simulink model "RADTRANS001"  (R2020b)
settings: Solver=VariableStepAuto  StartTime=0.0  StopTime=10.0  RelTol=1e-3
undefined symbols (not defined in the file): Line_110_C, Line_110_L, Line_110_R, Line_220_C, Line_220_L, Line_220_R, Line_35_C, Line_35_L, Line_35_R, Line_6_L, Line_6_R, Sys_f_Hz, Sys_V_net_kV, Tr_110_35_L_pu, Tr_110_35_R_pu, Tr_110_35_Sn_VA, Tr_110_35_V_HV_kV, Tr_110_35_V_LV_kV, Tr_110_6_L_pu, Tr_110_6_R_pu, Tr_110_6_Sn_VA, Tr_110_6_V_HV_kV, Tr_110_6_V_LV_kV, Tr_220_110_L_pu, Tr_220_110_R_pu, Tr_220_110_Sn_VA, Tr_220_110_V_HV_kV, Tr_220_110_V_LV_kV, Tr_35_04_L_pu, Tr_35_04_R_pu, Tr_35_04_Sn_VA, Tr_35_04_V_HV_kV, Tr_35_04_V_LV_kV, Tr_6_04_L_pu, Tr_6_04_R_pu, Tr_6_04_Sn_VA, Tr_6_04_V_HV_kV, Tr_6_04_V_LV_kV, Ts_powergui
libraries: dspstat3 x240, powerlib x169, powerlib_meascontrol x60
(part 6 of 6)

== system RADTRANS001/M_OUT_Завод_1_2 ==
  Iptg_4 : Display
      settings: Format=bank
  PQptg_4 : Scope  NumInputPorts=2
  "Power0 (3ph, Instantaneous)" : powerlib_meascontrol/Measurements/Power (3ph, Instantaneous)
  Pptg_4 : Display
      settings: Format=bank
  Qptg_4 : Display
      settings: Format=bank
  RMS0 : dspstat3/RMS  run=off  directionMode=Each column  dimension=1  InputProcessing=Columns as channels (frame based)  reset_popup=None
  RMS3 : dspstat3/RMS  run=off  directionMode=Each column  dimension=1  InputProcessing=Columns as channels (frame based)  reset_popup=None
  RMS4 : dspstat3/RMS  run=off  directionMode=Each column  dimension=1  InputProcessing=Columns as channels (frame based)  reset_popup=None
  RMSpt_4 : dspstat3/RMS  run=off  directionMode=Each column  dimension=1  InputProcessing=Columns as channels (frame based)  reset_popup=None
  Real-Ima to Complex : RealImagToComplex
  S : Abs
  SSptg_4 : Scope
  Sptg_4 : Display
      settings: Format=bank
  Three-Phase V-I Measurementpt_4 : powerlib/Measurements/Three-Phase V-I Measurement  VoltageMeasurement=phase-to-ground  SetLabelV=off  LabelV=Vabc  Vpu=off  VpuLL=off  CurrentMeasurement=yes  SetLabelI=off  LabelI=Iabc  Ipu=off  Pbase=100e6  Vbase=500e3  OutputType=Complex  PhasorSimulation=off  PSBequivalent=0
  UIptg_4 : Scope  NumInputPorts=2
  Uptg_4 : Display
      settings: Format=bank
  a : PMIOPort  Side=Right
  b : PMIOPort  Port=2  Side=Right
  c : PMIOPort  Port=3  Side=Right
  A : PMIOPort  Port=4  Side=Left
  B : PMIOPort  Port=5  Side=Left
  C : PMIOPort  Port=6  Side=Left
  tag scope: I_ptg_4=global, P_ptg_4=global, Q_ptg_4=global, S_ptg_4=global, U_ptg_4=global
  wires:
  S/1 -> [S_ptg_4]
  Real-Ima to Complex/1 -> S/1
  [S_ptg_4] -> Sptg_4/1
  [S_ptg_4] -> SSptg_4/1
  [P_ptg_4] -> RMSpt_4/1
  RMSpt_4/1 -> Pptg_4/1
  RMS0/1 -> Qptg_4/1
  [U_ptg_4] -> RMS3/1
  RMS3/1 -> Uptg_4/1
  [P_ptg_4] -> Real-Ima to Complex/1
  [Q_ptg_4] -> RMS0/1
  [I_ptg_4] -> RMS4/1
  RMS4/1 -> Iptg_4/1
  [U_ptg_4] -> UIptg_4/1  "U"
  [P_ptg_4] -> PQptg_4/1  "P"
  [I_ptg_4] -> UIptg_4/2  "I"
  Three-Phase V-I Measurementpt_4/1 -> [U_ptg_4]
  [Q_ptg_4] -> Real-Ima to Complex/2
  Three-Phase V-I Measurementpt_4/2 -> [I_ptg_4]
  [U_ptg_4] -> "Power0 (3ph, Instantaneous)"/1
  [I_ptg_4] -> "Power0 (3ph, Instantaneous)"/2
  "Power0 (3ph, Instantaneous)"/2 -> [Q_ptg_4]
  "Power0 (3ph, Instantaneous)"/1 -> [P_ptg_4]
  [Q_ptg_4] -> PQptg_4/2  "Q"
  connections:
  Three-Phase V-I Measurementpt_4/LConn1 -- A/RConn1
  Three-Phase V-I Measurementpt_4/RConn1 -- a/RConn1
  Three-Phase V-I Measurementpt_4/LConn2 -- B/RConn1
  Three-Phase V-I Measurementpt_4/LConn3 -- C/RConn1
  Three-Phase V-I Measurementpt_4/RConn3 -- c/RConn1
  Three-Phase V-I Measurementpt_4/RConn2 -- b/RConn1

== system RADTRANS001/M_OUT_Завод_2_1 ==
  Iptg_14 : Display
      settings: Format=bank
  PQptg_14 : Scope  NumInputPorts=2
  "Power0 (3ph, Instantaneous)" : powerlib_meascontrol/Measurements/Power (3ph, Instantaneous)
  Pptg_14 : Display
      settings: Format=bank
  Qptg_14 : Display
      settings: Format=bank
  RMS14 : dspstat3/RMS  run=off  directionMode=Each column  dimension=1  InputProcessing=Columns as channels (frame based)  reset_popup=None
  RMS3 : dspstat3/RMS  run=off  directionMode=Each column  dimension=1  InputProcessing=Columns as channels (frame based)  reset_popup=None
  RMS4 : dspstat3/RMS  run=off  directionMode=Each column  dimension=1  InputProcessing=Columns as channels (frame based)  reset_popup=None
  RMSpt_14 : dspstat3/RMS  run=off  directionMode=Each column  dimension=1  InputProcessing=Columns as channels (frame based)  reset_popup=None
  Real-Ima to Complex : RealImagToComplex
  S : Abs
  SSptg_14 : Scope
  Sptg_14 : Display
      settings: Format=bank
  Three-Phase V-I Measurementpt_14 : powerlib/Measurements/Three-Phase V-I Measurement  VoltageMeasurement=phase-to-ground  SetLabelV=off  LabelV=Vabc  Vpu=off  VpuLL=off  CurrentMeasurement=yes  SetLabelI=off  LabelI=Iabc  Ipu=off  Pbase=100e6  Vbase=500e3  OutputType=Complex  PhasorSimulation=off  PSBequivalent=0
  UIptg_14 : Scope  NumInputPorts=2
  Uptg_14 : Display
      settings: Format=bank
  a : PMIOPort  Side=Right
  b : PMIOPort  Port=2  Side=Right
  c : PMIOPort  Port=3  Side=Right
  A : PMIOPort  Port=4  Side=Left
  B : PMIOPort  Port=5  Side=Left
  C : PMIOPort  Port=6  Side=Left
  tag scope: I_ptg_14=global, P_ptg_14=global, Q_ptg_14=global, S_ptg_14=global, U_ptg_14=global
  wires:
  S/1 -> [S_ptg_14]
  Real-Ima to Complex/1 -> S/1
  [S_ptg_14] -> Sptg_14/1
  [S_ptg_14] -> SSptg_14/1
  [P_ptg_14] -> RMSpt_14/1
  RMSpt_14/1 -> Pptg_14/1
  RMS14/1 -> Qptg_14/1
  [U_ptg_14] -> RMS3/1
  RMS3/1 -> Uptg_14/1
  [P_ptg_14] -> Real-Ima to Complex/1
  [Q_ptg_14] -> RMS14/1
  [I_ptg_14] -> RMS4/1
  RMS4/1 -> Iptg_14/1
  [U_ptg_14] -> UIptg_14/1  "U"
  [P_ptg_14] -> PQptg_14/1  "P"
  [I_ptg_14] -> UIptg_14/2  "I"
  Three-Phase V-I Measurementpt_14/1 -> [U_ptg_14]
  [Q_ptg_14] -> Real-Ima to Complex/2
  Three-Phase V-I Measurementpt_14/2 -> [I_ptg_14]
  [U_ptg_14] -> "Power0 (3ph, Instantaneous)"/1
  [I_ptg_14] -> "Power0 (3ph, Instantaneous)"/2
  "Power0 (3ph, Instantaneous)"/2 -> [Q_ptg_14]
  "Power0 (3ph, Instantaneous)"/1 -> [P_ptg_14]
  [Q_ptg_14] -> PQptg_14/2  "Q"
  connections:
  Three-Phase V-I Measurementpt_14/LConn1 -- A/RConn1
  Three-Phase V-I Measurementpt_14/RConn1 -- a/RConn1
  Three-Phase V-I Measurementpt_14/LConn2 -- B/RConn1
  Three-Phase V-I Measurementpt_14/LConn3 -- C/RConn1
  Three-Phase V-I Measurementpt_14/RConn3 -- c/RConn1
  Three-Phase V-I Measurementpt_14/RConn2 -- b/RConn1

== system RADTRANS001/M_OUT_Завод_2_2 ==
  Iptg_16 : Display
      settings: Format=bank
  PQptg_16 : Scope  NumInputPorts=2
  "Power0 (3ph, Instantaneous)" : powerlib_meascontrol/Measurements/Power (3ph, Instantaneous)
  Pptg_16 : Display
      settings: Format=bank
  Qptg_16 : Display
      settings: Format=bank
  RMS16 : dspstat3/RMS  run=off  directionMode=Each column  dimension=1  InputProcessing=Columns as channels (frame based)  reset_popup=None
  RMS3 : dspstat3/RMS  run=off  directionMode=Each column  dimension=1  InputProcessing=Columns as channels (frame based)  reset_popup=None
  RMS4 : dspstat3/RMS  run=off  directionMode=Each column  dimension=1  InputProcessing=Columns as channels (frame based)  reset_popup=None
  RMSpt_16 : dspstat3/RMS  run=off  directionMode=Each column  dimension=1  InputProcessing=Columns as channels (frame based)  reset_popup=None
  Real-Ima to Complex : RealImagToComplex
  S : Abs
  SSptg_16 : Scope
  Sptg_16 : Display
      settings: Format=bank
  Three-Phase V-I Measurementpt_16 : powerlib/Measurements/Three-Phase V-I Measurement  VoltageMeasurement=phase-to-ground  SetLabelV=off  LabelV=Vabc  Vpu=off  VpuLL=off  CurrentMeasurement=yes  SetLabelI=off  LabelI=Iabc  Ipu=off  Pbase=100e6  Vbase=500e3  OutputType=Complex  PhasorSimulation=off  PSBequivalent=0
  UIptg_16 : Scope  NumInputPorts=2
  Uptg_16 : Display
      settings: Format=bank
  a : PMIOPort  Side=Right
  b : PMIOPort  Port=2  Side=Right
  c : PMIOPort  Port=3  Side=Right
  A : PMIOPort  Port=4  Side=Left
  B : PMIOPort  Port=5  Side=Left
  C : PMIOPort  Port=6  Side=Left
  tag scope: I_ptg_16=global, P_ptg_16=global, Q_ptg_16=global, S_ptg_16=global, U_ptg_16=global
  wires:
  S/1 -> [S_ptg_16]
  Real-Ima to Complex/1 -> S/1
  [S_ptg_16] -> Sptg_16/1
  [S_ptg_16] -> SSptg_16/1
  [P_ptg_16] -> RMSpt_16/1
  RMSpt_16/1 -> Pptg_16/1
  RMS16/1 -> Qptg_16/1
  [U_ptg_16] -> RMS3/1
  RMS3/1 -> Uptg_16/1
  [P_ptg_16] -> Real-Ima to Complex/1
  [Q_ptg_16] -> RMS16/1
  [I_ptg_16] -> RMS4/1
  RMS4/1 -> Iptg_16/1
  [U_ptg_16] -> UIptg_16/1  "U"
  [P_ptg_16] -> PQptg_16/1  "P"
  [I_ptg_16] -> UIptg_16/2  "I"
  Three-Phase V-I Measurementpt_16/1 -> [U_ptg_16]
  [Q_ptg_16] -> Real-Ima to Complex/2
  Three-Phase V-I Measurementpt_16/2 -> [I_ptg_16]
  [U_ptg_16] -> "Power0 (3ph, Instantaneous)"/1
  [I_ptg_16] -> "Power0 (3ph, Instantaneous)"/2
  "Power0 (3ph, Instantaneous)"/2 -> [Q_ptg_16]
  "Power0 (3ph, Instantaneous)"/1 -> [P_ptg_16]
  [Q_ptg_16] -> PQptg_16/2  "Q"
  connections:
  Three-Phase V-I Measurementpt_16/LConn1 -- A/RConn1
  Three-Phase V-I Measurementpt_16/RConn1 -- a/RConn1
  Three-Phase V-I Measurementpt_16/LConn2 -- B/RConn1
  Three-Phase V-I Measurementpt_16/LConn3 -- C/RConn1
  Three-Phase V-I Measurementpt_16/RConn3 -- c/RConn1
  Three-Phase V-I Measurementpt_16/RConn2 -- b/RConn1

== system RADTRANS001/M_OUT_Завод_3_1 ==
  Iptg_26 : Display
      settings: Format=bank
  PQptg_26 : Scope  NumInputPorts=2
  "Power0 (3ph, Instantaneous)" : powerlib_meascontrol/Measurements/Power (3ph, Instantaneous)
  Pptg_26 : Display
      settings: Format=bank
  Qptg_26 : Display
      settings: Format=bank
  RMS26 : dspstat3/RMS  run=off  directionMode=Each column  dimension=1  InputProcessing=Columns as channels (frame based)  reset_popup=None
  RMS3 : dspstat3/RMS  run=off  directionMode=Each column  dimension=1  InputProcessing=Columns as channels (frame based)  reset_popup=None
  RMS4 : dspstat3/RMS  run=off  directionMode=Each column  dimension=1  InputProcessing=Columns as channels (frame based)  reset_popup=None
  RMSpt_26 : dspstat3/RMS  run=off  directionMode=Each column  dimension=1  InputProcessing=Columns as channels (frame based)  reset_popup=None
  Real-Ima to Complex : RealImagToComplex
  S : Abs
  SSptg_26 : Scope
  Sptg_26 : Display
      settings: Format=bank
  Three-Phase V-I Measurementpt_26 : powerlib/Measurements/Three-Phase V-I Measurement  VoltageMeasurement=phase-to-ground  SetLabelV=off  LabelV=Vabc  Vpu=off  VpuLL=off  CurrentMeasurement=yes  SetLabelI=off  LabelI=Iabc  Ipu=off  Pbase=100e6  Vbase=500e3  OutputType=Complex  PhasorSimulation=off  PSBequivalent=0
  UIptg_26 : Scope  NumInputPorts=2
  Uptg_26 : Display
      settings: Format=bank
  a : PMIOPort  Side=Right
  b : PMIOPort  Port=2  Side=Right
  c : PMIOPort  Port=3  Side=Right
  A : PMIOPort  Port=4  Side=Left
  B : PMIOPort  Port=5  Side=Left
  C : PMIOPort  Port=6  Side=Left
  tag scope: I_ptg_26=global, P_ptg_26=global, Q_ptg_26=global, S_ptg_26=global, U_ptg_26=global
  wires:
  S/1 -> [S_ptg_26]
  Real-Ima to Complex/1 -> S/1
  [S_ptg_26] -> Sptg_26/1
  [S_ptg_26] -> SSptg_26/1
  [P_ptg_26] -> RMSpt_26/1
  RMSpt_26/1 -> Pptg_26/1
  RMS26/1 -> Qptg_26/1
  [U_ptg_26] -> RMS3/1
  RMS3/1 -> Uptg_26/1
  [P_ptg_26] -> Real-Ima to Complex/1
  [Q_ptg_26] -> RMS26/1
  [I_ptg_26] -> RMS4/1
  RMS4/1 -> Iptg_26/1
  [U_ptg_26] -> UIptg_26/1  "U"
  [P_ptg_26] -> PQptg_26/1  "P"
  [I_ptg_26] -> UIptg_26/2  "I"
  Three-Phase V-I Measurementpt_26/1 -> [U_ptg_26]
  [Q_ptg_26] -> Real-Ima to Complex/2
  Three-Phase V-I Measurementpt_26/2 -> [I_ptg_26]
  [U_ptg_26] -> "Power0 (3ph, Instantaneous)"/1
  [I_ptg_26] -> "Power0 (3ph, Instantaneous)"/2
  "Power0 (3ph, Instantaneous)"/2 -> [Q_ptg_26]
  "Power0 (3ph, Instantaneous)"/1 -> [P_ptg_26]
  [Q_ptg_26] -> PQptg_26/2  "Q"
  connections:
  Three-Phase V-I Measurementpt_26/LConn1 -- A/RConn1
  Three-Phase V-I Measurementpt_26/RConn1 -- a/RConn1
  Three-Phase V-I Measurementpt_26/LConn2 -- B/RConn1
  Three-Phase V-I Measurementpt_26/LConn3 -- C/RConn1
  Three-Phase V-I Measurementpt_26/RConn3 -- c/RConn1
  Three-Phase V-I Measurementpt_26/RConn2 -- b/RConn1

== system RADTRANS001/M_OUT_Завод_3_2 ==
  Iptg_28 : Display
      settings: Format=bank
  PQptg_28 : Scope  NumInputPorts=2
  "Power0 (3ph, Instantaneous)" : powerlib_meascontrol/Measurements/Power (3ph, Instantaneous)
  Pptg_28 : Display
      settings: Format=bank
  Qptg_28 : Display
      settings: Format=bank
  RMS28 : dspstat3/RMS  run=off  directionMode=Each column  dimension=1  InputProcessing=Columns as channels (frame based)  reset_popup=None
  RMS3 : dspstat3/RMS  run=off  directionMode=Each column  dimension=1  InputProcessing=Columns as channels (frame based)  reset_popup=None
  RMS4 : dspstat3/RMS  run=off  directionMode=Each column  dimension=1  InputProcessing=Columns as channels (frame based)  reset_popup=None
  RMSpt_28 : dspstat3/RMS  run=off  directionMode=Each column  dimension=1  InputProcessing=Columns as channels (frame based)  reset_popup=None
  Real-Ima to Complex : RealImagToComplex
  S : Abs
  SSptg_28 : Scope
  Sptg_28 : Display
      settings: Format=bank
  Three-Phase V-I Measurementpt_28 : powerlib/Measurements/Three-Phase V-I Measurement  VoltageMeasurement=phase-to-ground  SetLabelV=off  LabelV=Vabc  Vpu=off  VpuLL=off  CurrentMeasurement=yes  SetLabelI=off  LabelI=Iabc  Ipu=off  Pbase=100e6  Vbase=500e3  OutputType=Complex  PhasorSimulation=off  PSBequivalent=0
  UIptg_28 : Scope  NumInputPorts=2
  Uptg_28 : Display
      settings: Format=bank
  a : PMIOPort  Side=Right
  b : PMIOPort  Port=2  Side=Right
  c : PMIOPort  Port=3  Side=Right
  A : PMIOPort  Port=4  Side=Left
  B : PMIOPort  Port=5  Side=Left
  C : PMIOPort  Port=6  Side=Left
  tag scope: I_ptg_28=global, P_ptg_28=global, Q_ptg_28=global, S_ptg_28=global, U_ptg_28=global
  wires:
  S/1 -> [S_ptg_28]
  Real-Ima to Complex/1 -> S/1
  [S_ptg_28] -> Sptg_28/1
  [S_ptg_28] -> SSptg_28/1
  [P_ptg_28] -> RMSpt_28/1
  RMSpt_28/1 -> Pptg_28/1
  RMS28/1 -> Qptg_28/1
  [U_ptg_28] -> RMS3/1
  RMS3/1 -> Uptg_28/1
  [P_ptg_28] -> Real-Ima to Complex/1
  [Q_ptg_28] -> RMS28/1
  [I_ptg_28] -> RMS4/1
  RMS4/1 -> Iptg_28/1
  [U_ptg_28] -> UIptg_28/1  "U"
  [P_ptg_28] -> PQptg_28/1  "P"
  [I_ptg_28] -> UIptg_28/2  "I"
  Three-Phase V-I Measurementpt_28/1 -> [U_ptg_28]
  [Q_ptg_28] -> Real-Ima to Complex/2
  Three-Phase V-I Measurementpt_28/2 -> [I_ptg_28]
  [U_ptg_28] -> "Power0 (3ph, Instantaneous)"/1
  [I_ptg_28] -> "Power0 (3ph, Instantaneous)"/2
  "Power0 (3ph, Instantaneous)"/2 -> [Q_ptg_28]
  "Power0 (3ph, Instantaneous)"/1 -> [P_ptg_28]
  [Q_ptg_28] -> PQptg_28/2  "Q"
  connections:
  Three-Phase V-I Measurementpt_28/LConn1 -- A/RConn1
  Three-Phase V-I Measurementpt_28/RConn1 -- a/RConn1
  Three-Phase V-I Measurementpt_28/LConn2 -- B/RConn1
  Three-Phase V-I Measurementpt_28/LConn3 -- C/RConn1
  Three-Phase V-I Measurementpt_28/RConn3 -- c/RConn1
  Three-Phase V-I Measurementpt_28/RConn2 -- b/RConn1

== system RADTRANS001/M_OUT_Завод_4_1 ==
  Iptg_38 : Display
      settings: Format=bank
  PQptg_38 : Scope  NumInputPorts=2
  "Power0 (3ph, Instantaneous)" : powerlib_meascontrol/Measurements/Power (3ph, Instantaneous)
  Pptg_38 : Display
      settings: Format=bank
  Qptg_38 : Display
      settings: Format=bank
  RMS3 : dspstat3/RMS  run=off  directionMode=Each column  dimension=1  InputProcessing=Columns as channels (frame based)  reset_popup=None
  RMS38 : dspstat3/RMS  run=off  directionMode=Each column  dimension=1  InputProcessing=Columns as channels (frame based)  reset_popup=None
  RMS4 : dspstat3/RMS  run=off  directionMode=Each column  dimension=1  InputProcessing=Columns as channels (frame based)  reset_popup=None
  RMSpt_38 : dspstat3/RMS  run=off  directionMode=Each column  dimension=1  InputProcessing=Columns as channels (frame based)  reset_popup=None
  Real-Ima to Complex : RealImagToComplex
  S : Abs
  SSptg_38 : Scope
  Sptg_38 : Display
      settings: Format=bank
  Three-Phase V-I Measurementpt_38 : powerlib/Measurements/Three-Phase V-I Measurement  VoltageMeasurement=phase-to-ground  SetLabelV=off  LabelV=Vabc  Vpu=off  VpuLL=off  CurrentMeasurement=yes  SetLabelI=off  LabelI=Iabc  Ipu=off  Pbase=100e6  Vbase=500e3  OutputType=Complex  PhasorSimulation=off  PSBequivalent=0
  UIptg_38 : Scope  NumInputPorts=2
  Uptg_38 : Display
      settings: Format=bank
  a : PMIOPort  Side=Right
  b : PMIOPort  Port=2  Side=Right
  c : PMIOPort  Port=3  Side=Right
  A : PMIOPort  Port=4  Side=Left
  B : PMIOPort  Port=5  Side=Left
  C : PMIOPort  Port=6  Side=Left
  tag scope: I_ptg_38=global, P_ptg_38=global, Q_ptg_38=global, S_ptg_38=global, U_ptg_38=global
  wires:
  S/1 -> [S_ptg_38]
  Real-Ima to Complex/1 -> S/1
  [S_ptg_38] -> Sptg_38/1
  [S_ptg_38] -> SSptg_38/1
  [P_ptg_38] -> RMSpt_38/1
  RMSpt_38/1 -> Pptg_38/1
  RMS38/1 -> Qptg_38/1
  [U_ptg_38] -> RMS3/1
  RMS3/1 -> Uptg_38/1
  [P_ptg_38] -> Real-Ima to Complex/1
  [Q_ptg_38] -> RMS38/1
  [I_ptg_38] -> RMS4/1
  RMS4/1 -> Iptg_38/1
  [U_ptg_38] -> UIptg_38/1  "U"
  [P_ptg_38] -> PQptg_38/1  "P"
  [I_ptg_38] -> UIptg_38/2  "I"
  Three-Phase V-I Measurementpt_38/1 -> [U_ptg_38]
  [Q_ptg_38] -> Real-Ima to Complex/2
  Three-Phase V-I Measurementpt_38/2 -> [I_ptg_38]
  [U_ptg_38] -> "Power0 (3ph, Instantaneous)"/1
  [I_ptg_38] -> "Power0 (3ph, Instantaneous)"/2
  "Power0 (3ph, Instantaneous)"/2 -> [Q_ptg_38]
  "Power0 (3ph, Instantaneous)"/1 -> [P_ptg_38]
  [Q_ptg_38] -> PQptg_38/2  "Q"
  connections:
  Three-Phase V-I Measurementpt_38/LConn1 -- A/RConn1
  Three-Phase V-I Measurementpt_38/RConn1 -- a/RConn1
  Three-Phase V-I Measurementpt_38/LConn2 -- B/RConn1
  Three-Phase V-I Measurementpt_38/LConn3 -- C/RConn1
  Three-Phase V-I Measurementpt_38/RConn3 -- c/RConn1
  Three-Phase V-I Measurementpt_38/RConn2 -- b/RConn1

== system RADTRANS001/M_OUT_Завод_4_2 ==
  Iptg_40 : Display
      settings: Format=bank
  PQptg_40 : Scope  NumInputPorts=2
  "Power0 (3ph, Instantaneous)" : powerlib_meascontrol/Measurements/Power (3ph, Instantaneous)
  Pptg_40 : Display
      settings: Format=bank
  Qptg_40 : Display
      settings: Format=bank
  RMS3 : dspstat3/RMS  run=off  directionMode=Each column  dimension=1  InputProcessing=Columns as channels (frame based)  reset_popup=None
  RMS4 : dspstat3/RMS  run=off  directionMode=Each column  dimension=1  InputProcessing=Columns as channels (frame based)  reset_popup=None
  RMS40 : dspstat3/RMS  run=off  directionMode=Each column  dimension=1  InputProcessing=Columns as channels (frame based)  reset_popup=None
  RMSpt_40 : dspstat3/RMS  run=off  directionMode=Each column  dimension=1  InputProcessing=Columns as channels (frame based)  reset_popup=None
  Real-Ima to Complex : RealImagToComplex
  S : Abs
  SSptg_40 : Scope
  Sptg_40 : Display
      settings: Format=bank
  Three-Phase V-I Measurementpt_40 : powerlib/Measurements/Three-Phase V-I Measurement  VoltageMeasurement=phase-to-ground  SetLabelV=off  LabelV=Vabc  Vpu=off  VpuLL=off  CurrentMeasurement=yes  SetLabelI=off  LabelI=Iabc  Ipu=off  Pbase=100e6  Vbase=500e3  OutputType=Complex  PhasorSimulation=off  PSBequivalent=0
  UIptg_40 : Scope  NumInputPorts=2
  Uptg_40 : Display
      settings: Format=bank
  a : PMIOPort  Side=Right
  b : PMIOPort  Port=2  Side=Right
  c : PMIOPort  Port=3  Side=Right
  A : PMIOPort  Port=4  Side=Left
  B : PMIOPort  Port=5  Side=Left
  C : PMIOPort  Port=6  Side=Left
  tag scope: I_ptg_40=global, P_ptg_40=global, Q_ptg_40=global, S_ptg_40=global, U_ptg_40=global
  wires:
  S/1 -> [S_ptg_40]
  Real-Ima to Complex/1 -> S/1
  [S_ptg_40] -> Sptg_40/1
  [S_ptg_40] -> SSptg_40/1
  [P_ptg_40] -> RMSpt_40/1
  RMSpt_40/1 -> Pptg_40/1
  RMS40/1 -> Qptg_40/1
  [U_ptg_40] -> RMS3/1
  RMS3/1 -> Uptg_40/1
  [P_ptg_40] -> Real-Ima to Complex/1
  [Q_ptg_40] -> RMS40/1
  [I_ptg_40] -> RMS4/1
  RMS4/1 -> Iptg_40/1
  [U_ptg_40] -> UIptg_40/1  "U"
  [P_ptg_40] -> PQptg_40/1  "P"
  [I_ptg_40] -> UIptg_40/2  "I"
  Three-Phase V-I Measurementpt_40/1 -> [U_ptg_40]
  [Q_ptg_40] -> Real-Ima to Complex/2
  Three-Phase V-I Measurementpt_40/2 -> [I_ptg_40]
  [U_ptg_40] -> "Power0 (3ph, Instantaneous)"/1
  [I_ptg_40] -> "Power0 (3ph, Instantaneous)"/2
  "Power0 (3ph, Instantaneous)"/2 -> [Q_ptg_40]
  "Power0 (3ph, Instantaneous)"/1 -> [P_ptg_40]
  [Q_ptg_40] -> PQptg_40/2  "Q"
  connections:
  Three-Phase V-I Measurementpt_40/LConn1 -- A/RConn1
  Three-Phase V-I Measurementpt_40/RConn1 -- a/RConn1
  Three-Phase V-I Measurementpt_40/LConn2 -- B/RConn1
  Three-Phase V-I Measurementpt_40/LConn3 -- C/RConn1
  Three-Phase V-I Measurementpt_40/RConn3 -- c/RConn1
  Three-Phase V-I Measurementpt_40/RConn2 -- b/RConn1

== system RADTRANS001/M_OUT_Завод_5_1 ==
  Iptg_50 : Display
      settings: Format=bank
  PQptg_50 : Scope  NumInputPorts=2
  "Power0 (3ph, Instantaneous)" : powerlib_meascontrol/Measurements/Power (3ph, Instantaneous)
  Pptg_50 : Display
      settings: Format=bank
  Qptg_50 : Display
      settings: Format=bank
  RMS3 : dspstat3/RMS  run=off  directionMode=Each column  dimension=1  InputProcessing=Columns as channels (frame based)  reset_popup=None
  RMS4 : dspstat3/RMS  run=off  directionMode=Each column  dimension=1  InputProcessing=Columns as channels (frame based)  reset_popup=None
  RMS50 : dspstat3/RMS  run=off  directionMode=Each column  dimension=1  InputProcessing=Columns as channels (frame based)  reset_popup=None
  RMSpt_50 : dspstat3/RMS  run=off  directionMode=Each column  dimension=1  InputProcessing=Columns as channels (frame based)  reset_popup=None
  Real-Ima to Complex : RealImagToComplex
  S : Abs
  SSptg_50 : Scope
  Sptg_50 : Display
      settings: Format=bank
  Three-Phase V-I Measurementpt_50 : powerlib/Measurements/Three-Phase V-I Measurement  VoltageMeasurement=phase-to-ground  SetLabelV=off  LabelV=Vabc  Vpu=off  VpuLL=off  CurrentMeasurement=yes  SetLabelI=off  LabelI=Iabc  Ipu=off  Pbase=100e6  Vbase=500e3  OutputType=Complex  PhasorSimulation=off  PSBequivalent=0
  UIptg_50 : Scope  NumInputPorts=2
  Uptg_50 : Display
      settings: Format=bank
  a : PMIOPort  Side=Right
  b : PMIOPort  Port=2  Side=Right
  c : PMIOPort  Port=3  Side=Right
  A : PMIOPort  Port=4  Side=Left
  B : PMIOPort  Port=5  Side=Left
  C : PMIOPort  Port=6  Side=Left
  tag scope: I_ptg_50=global, P_ptg_50=global, Q_ptg_50=global, S_ptg_50=global, U_ptg_50=global
  wires:
  S/1 -> [S_ptg_50]
  Real-Ima to Complex/1 -> S/1
  [S_ptg_50] -> Sptg_50/1
  [S_ptg_50] -> SSptg_50/1
  [P_ptg_50] -> RMSpt_50/1
  RMSpt_50/1 -> Pptg_50/1
  RMS50/1 -> Qptg_50/1
  [U_ptg_50] -> RMS3/1
  RMS3/1 -> Uptg_50/1
  [P_ptg_50] -> Real-Ima to Complex/1
  [Q_ptg_50] -> RMS50/1
  [I_ptg_50] -> RMS4/1
  RMS4/1 -> Iptg_50/1
  [U_ptg_50] -> UIptg_50/1  "U"
  [P_ptg_50] -> PQptg_50/1  "P"
  [I_ptg_50] -> UIptg_50/2  "I"
  Three-Phase V-I Measurementpt_50/1 -> [U_ptg_50]
  [Q_ptg_50] -> Real-Ima to Complex/2
  Three-Phase V-I Measurementpt_50/2 -> [I_ptg_50]
  [U_ptg_50] -> "Power0 (3ph, Instantaneous)"/1
  [I_ptg_50] -> "Power0 (3ph, Instantaneous)"/2
  "Power0 (3ph, Instantaneous)"/2 -> [Q_ptg_50]
  "Power0 (3ph, Instantaneous)"/1 -> [P_ptg_50]
  [Q_ptg_50] -> PQptg_50/2  "Q"
  connections:
  Three-Phase V-I Measurementpt_50/LConn1 -- A/RConn1
  Three-Phase V-I Measurementpt_50/RConn1 -- a/RConn1
  Three-Phase V-I Measurementpt_50/LConn2 -- B/RConn1
  Three-Phase V-I Measurementpt_50/LConn3 -- C/RConn1
  Three-Phase V-I Measurementpt_50/RConn3 -- c/RConn1
  Three-Phase V-I Measurementpt_50/RConn2 -- b/RConn1

== system RADTRANS001/M_OUT_Завод_5_2 ==
  Iptg_52 : Display
      settings: Format=bank
  PQptg_52 : Scope  NumInputPorts=2
  "Power0 (3ph, Instantaneous)" : powerlib_meascontrol/Measurements/Power (3ph, Instantaneous)
  Pptg_52 : Display
      settings: Format=bank
  Qptg_52 : Display
      settings: Format=bank
  RMS3 : dspstat3/RMS  run=off  directionMode=Each column  dimension=1  InputProcessing=Columns as channels (frame based)  reset_popup=None
  RMS4 : dspstat3/RMS  run=off  directionMode=Each column  dimension=1  InputProcessing=Columns as channels (frame based)  reset_popup=None
  RMS52 : dspstat3/RMS  run=off  directionMode=Each column  dimension=1  InputProcessing=Columns as channels (frame based)  reset_popup=None
  RMSpt_52 : dspstat3/RMS  run=off  directionMode=Each column  dimension=1  InputProcessing=Columns as channels (frame based)  reset_popup=None
  Real-Ima to Complex : RealImagToComplex
  S : Abs
  SSptg_52 : Scope
  Sptg_52 : Display
      settings: Format=bank
  Three-Phase V-I Measurementpt_52 : powerlib/Measurements/Three-Phase V-I Measurement  VoltageMeasurement=phase-to-ground  SetLabelV=off  LabelV=Vabc  Vpu=off  VpuLL=off  CurrentMeasurement=yes  SetLabelI=off  LabelI=Iabc  Ipu=off  Pbase=100e6  Vbase=500e3  OutputType=Complex  PhasorSimulation=off  PSBequivalent=0
  UIptg_52 : Scope  NumInputPorts=2
  Uptg_52 : Display
      settings: Format=bank
  a : PMIOPort  Side=Right
  b : PMIOPort  Port=2  Side=Right
  c : PMIOPort  Port=3  Side=Right
  A : PMIOPort  Port=4  Side=Left
  B : PMIOPort  Port=5  Side=Left
  C : PMIOPort  Port=6  Side=Left
  tag scope: I_ptg_52=global, P_ptg_52=global, Q_ptg_52=global, S_ptg_52=global, U_ptg_52=global
  wires:
  S/1 -> [S_ptg_52]
  Real-Ima to Complex/1 -> S/1
  [S_ptg_52] -> Sptg_52/1
  [S_ptg_52] -> SSptg_52/1
  [P_ptg_52] -> RMSpt_52/1
  RMSpt_52/1 -> Pptg_52/1
  RMS52/1 -> Qptg_52/1
  [U_ptg_52] -> RMS3/1
  RMS3/1 -> Uptg_52/1
  [P_ptg_52] -> Real-Ima to Complex/1
  [Q_ptg_52] -> RMS52/1
  [I_ptg_52] -> RMS4/1
  RMS4/1 -> Iptg_52/1
  [U_ptg_52] -> UIptg_52/1  "U"
  [P_ptg_52] -> PQptg_52/1  "P"
  [I_ptg_52] -> UIptg_52/2  "I"
  Three-Phase V-I Measurementpt_52/1 -> [U_ptg_52]
  [Q_ptg_52] -> Real-Ima to Complex/2
  Three-Phase V-I Measurementpt_52/2 -> [I_ptg_52]
  [U_ptg_52] -> "Power0 (3ph, Instantaneous)"/1
  [I_ptg_52] -> "Power0 (3ph, Instantaneous)"/2
  "Power0 (3ph, Instantaneous)"/2 -> [Q_ptg_52]
  "Power0 (3ph, Instantaneous)"/1 -> [P_ptg_52]
  [Q_ptg_52] -> PQptg_52/2  "Q"
  connections:
  Three-Phase V-I Measurementpt_52/LConn1 -- A/RConn1
  Three-Phase V-I Measurementpt_52/RConn1 -- a/RConn1
  Three-Phase V-I Measurementpt_52/LConn2 -- B/RConn1
  Three-Phase V-I Measurementpt_52/LConn3 -- C/RConn1
  Three-Phase V-I Measurementpt_52/RConn3 -- c/RConn1
  Three-Phase V-I Measurementpt_52/RConn2 -- b/RConn1
